simulink model "Kal_6Dpitch_sim"  (R2023b)
settings: Solver=FixedStepAuto  StartTime=0.0  StopTime=30  FixedStep=0.001  RelTol=1e-3
values from neighbouring files (symbols this model uses):
  beta = pi/10    (= 0.314159265359)    [Kal_6Dpitch_mat.m]    (also in TestValori.m = -0.628318530718; TestVel.m = 0.523598775598)
  cov_ic = [10, 0 ... (first row only)    [KalPrep_mat.m]    (also in Kal_6Dpitch_mat.m = cov_ic * (1 + 2*rand); Kal_pitch_mat.m = cov_ic * (1 + 2*rand))
  des_vel = [0.1, 0, 0, 0]'    [Kal_6Dpitch_mat.m]    (also in Los_path_mat.m)
  eta1 = deg2rad(1)    [KalPrep_mat.m]    (also in Kal_6Dpitch_mat.m = 0.05; Kal_pitch_mat.m = 0.15)
  eta2 = 0.05    [Kal_6Dpitch_mat.m]    (also in Kal_pitch_mat.m = 0.2)
  G = [Ts 0 ... (first row only)    [KalPrep_mat.m]    (also in Kal_6Dpitch_mat.m = eye(3) * Ts; Kal_pitch_mat.m = eye(3) * Ts)
  Gamma = -pi/6    (= -0.523598775598)    [Kal_6Dpitch_mat.m]    (also in TestValori.m)
  h_ref = 7    [Kal_6Dpitch_mat.m]
  init_cond = [pi/2; 5]    [KalPrep_mat.m]    (also in Kal_6Dpitch_mat.m = [2; 0; 0]; Kal_pitch_mat.m = [0; 0; 0])
  Kd_dep = (p + 2*damp*wn)*mv(3) + dv(3)    [Control_gains_mat.m]    (also in Los_path_mat.m = (p + 2*damp*wn)*mv(4) + dv(4))
  Ki_dep = p*(wn^2)*mv(3)    [Control_gains_mat.m]    (also in Los_path_mat.m = p*(wn^2)*mv(4))
  Ki_surge = wn^2 * mv(1)    [Control_gains_mat.m]    (also in Los_path_mat.m)
  Kp_dep = mv(3)*((wn^2) + 2*damp*p*wn)    [Control_gains_mat.m]    (also in Los_path_mat.m = mv(4)*((wn^2) + 2*damp*p*wn))
  Kp_surge = 2*damp*wn*mv(1) - dv(1)    [Control_gains_mat.m]    (also in Los_path_mat.m)
  Kt_dep = 1 / sqrt(ti_dep*td_dep)    [Control_gains_mat.m]
  Kt_surge = 1 / ti_surge    [Control_gains_mat.m]
  Lambda = pi/6    (= 0.523598775598)    [Kal_6Dpitch_mat.m]    (also in TestValori.m)
  pr0 = [0,0]'    [Kal_6Dpitch_mat.m]
  Q = [(sig1^2), 0 ... (first row only)    [KalPrep_mat.m]    (also in Kal_6Dpitch_mat.m = zeros(3,3); Kal_pitch_mat.m = zeros(3,3))
  qt = - 10    (= -10)    [Kal_6Dpitch_mat.m]    (also in TestValori.m = -5)
  R = (eta1)^2    [KalPrep_mat.m]    (also in Kal_6Dpitch_mat.m = [(eta1^2), 0; Kal_pitch_mat.m = [eta1, 0; untitled.m = 10)
  sat_dep = 15    [Model_6Deq_mat.m]
  sat_surge = 15    [Model_6Deq_mat.m]
  sat_tr = 2000    [Model_6Deq_mat.m]
  sig1 = 0.1    [KalPrep_mat.m]    (also in Kal_6Dpitch_mat.m; Kal_pitch_mat.m)
  sig2 = 0.2    [KalPrep_mat.m]    (also in Kal_6Dpitch_mat.m; Kal_pitch_mat.m)
  sig3 = 0.15    [Kal_6Dpitch_mat.m]    (also in Kal_pitch_mat.m)
  speed0 = [0.1, 0, 0, 0]'    [Los_path_mat.m]    (also in Model_6Deq_mat.m = [0.1, 0, 0, 0, 0, 0]')
  Ts = 0.001    [KalPrep_mat.m]    (also in Kal_6Dpitch_mat.m; Kal_pitch_mat.m; TestVel.m)
undefined symbols (not defined in the file or in its folder): Kd_theta, Ki_theta, Kp_theta, Kt_theta
settings Model: NumberOfSteps=100  SnapshotInterval=1000  Creator=fabio  LastModifiedBy=fabio

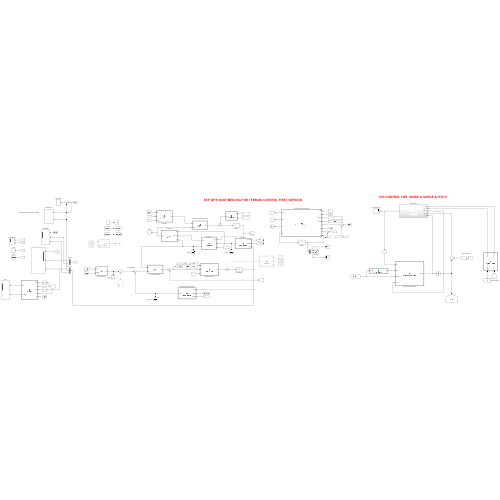
[thumbnail: Simulink's stored preview of the top-level diagram]
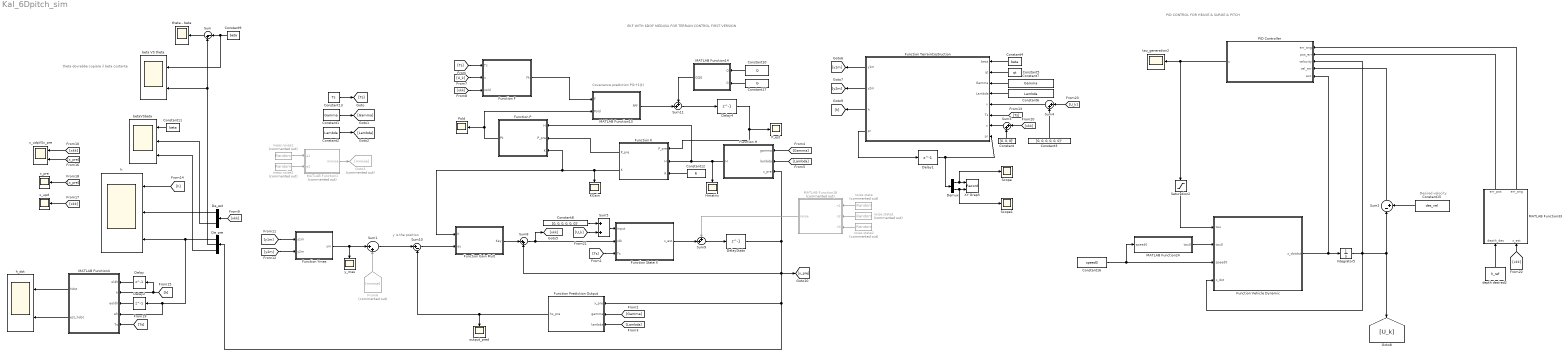
== system Kal_6Dpitch_sim ==
  note: theta dovrebbe copiare il beta costante
  note: Covariance prediction P(k+1|k)
  note: EKF WITH 6DOF MEDUSA FOR TERRAIN CONTROL FIRST VERSION
  note: y is the position
  note: PID CONTROL FOR HEAVE & SURGE & PITCH
  note: Desired velocity
  Constant : Constant  Value=[0, 0, 0]'
  Constant1 : Constant  Value=Gamma
  Constant10 : Constant  Value=Q  VectorParams1D=off
  Constant11 : Constant  Value=beta
  Constant12 : Constant  Value=R
  Constant13 : Constant  Value=Ts
  Constant15 : Constant  Value=des_vel
  Constant16 : Constant  Value=speed0
  Constant17 : Constant  Value=G  VectorParams1D=off
  Constant2 : Constant  Value=Lambda
  Constant3 : Constant  Value=[0, 0, 0, 0, 0, 0]'
  Constant4 : Constant  Value=beta
  Constant5 : Constant  Value=qt
  Constant6 : Constant  Value=Lambda
  Constant7 : Constant  Value=Gamma
  Constant8 : Constant  Value=[0, 0, 0, 0, 0, 0]'
  Constant9 : Constant  Value=beta
  De_est : Demux  Outputs=3
  De_pre : Demux  Outputs=3
  Delay : Delay  DelayLength=1
  Delay1 : Delay  DelayLength=1  InitialCondition=pr0  UseCircularBuffer=on
  Delay2 : Delay  DelayLength=1
  Delay4 : Delay  DelayLength=1  InitialCondition=cov_ic  UseCircularBuffer=on
  DelayStato : Delay  DelayLength=1  InitialCondition=init_cond  UseCircularBuffer=on
  Demux : Demux  Outputs=2
  From6 : From  Commented=on  GotoTag=mnoise
  Function F : MATLAB Function  TreatAsAtomicUnit=on
  Function Gain Mult : MATLAB Function  TreatAsAtomicUnit=on
  Function H : MATLAB Function  TreatAsAtomicUnit=on
  Function K : MATLAB Function  TreatAsAtomicUnit=on
  Function P : MATLAB Function  TreatAsAtomicUnit=on
  Function Prediction Output : MATLAB Function  TreatAsAtomicUnit=on
  Function State X : MATLAB Function  TreatAsAtomicUnit=on
  Function TerrainCostruction : MATLAB Function  TreatAsAtomicUnit=on
  Function Vehicle Dynamic : MATLAB Function  TreatAsAtomicUnit=on
  Function Ymes : MATLAB Function  TreatAsAtomicUnit=on
  Goto3 : Goto  Commented=on  GotoTag=mnoise
  Hmatrix : Scope
  Integrator5 : Integrator
  KGain : Scope
  MATLAB Function1 : MATLAB Function  Commented=on  TreatAsAtomicUnit=on
  MATLAB Function13 : MATLAB Function  TreatAsAtomicUnit=on
  MATLAB Function14 : MATLAB Function  TreatAsAtomicUnit=on
  MATLAB Function18 : MATLAB Function  Commented=on  TreatAsAtomicUnit=on
  MATLAB Function24 : MATLAB Function  TreatAsAtomicUnit=on
  MATLAB Function33 : MATLAB Function  TreatAsAtomicUnit=on
  MATLAB Function4 : MATLAB Function  TreatAsAtomicUnit=on
  PID Controller : Subsystem
  P_est : Scope
  Pold : Scope
  Saturation2 : Saturate  UpperLimit=sat_tr  LowerLimit=-sat_tr
  Scope : Scope
  Scope1 : Scope
  Sum : Sum  Inputs=|-+
  Sum{1,3..4,8} (4 alike) : Sum  Inputs=|++
  Sum10 : Sum  Inputs=|+-
  Sum11 : Sum  Inputs=++|
  Sum2 : Sum  Inputs=|-+
  Sum5 : Sum
  Sum9 : Sum  Inputs=++|
  XY Graph : Record  FileSettingsInternal="{\"entries\":[{\"content\":{\"excelSettings\":{\"content\":{},\"type\":\"Streamout.ExcelSettings\"}},\"type\":\"Streamout.FileSettingStorage\",\"uuid\":\"\"}],\"packageUris\":[\"http:\\/\\/schema.mathworks.com\\/mf0\\/streamout_blocks\\/R2020a\"],\"version\":\"1.0\"}"  Layout=[1 1]  SignalsInternal="{\"entries\":[{\"content\":{\"signals\":[{\"content\":{\"blockPath\":[],\"dimensions\":[1],\"domain\":\"\",\"lineColor\":\"#a2142f\",\"plots\":[ 1 ],\"port\":1,\"signalID\":1,\"signalName\":\"Demux:1\"},\"type\":\"RecordBlkView.Signal\",\"uuid\":\"\"},{\"content\":{\"blockPath\":[],\"dimensions\":[1],\"domain\":\"\",\"lineColor\":\"#139fff\",\"plots\":[ 1 ],\"port\":2,\"signalID\":2,\"signalName\":\"Demux:2\"},\"type\":\"RecordBlkView.Signal\",\"uuid\":\"\"}]},\"type\":\"RecordBlkView.InputSignals\",\"uuid\":\"\"}],\"packageUris\":[\"http:\\/\\/schema.mathworks.com\\/mf0\\/streamout_blocks\\/R2020a\"],\"version\":\"1.0\"}"  VisualizationBindings="{\"xyplotplugin\":{\"info\":[{\"series\":[{\"bindingParametersList\":[{\"parameter\":\"X-Axis\",\"signalID\":1,\"signalName\":\"Demux:1\"},{\"parameter\":\"Y-Axis\",\"signalID\":2,\"signalName\":\"Demux:2\"}],\"seriesID\":0}],\"subplotID\":1}]}}"  CompatibilityTag=XY
  beta VS theta : Scope  NumInputPorts=2
  betaVSbeta : Scope  NumInputPorts=3
  depth desired2 : Constant  Value=h_ref
  h : Scope  NumInputPorts=3
  h_dot : Scope  NumInputPorts=2
  meas.noise1 : RandomNumber  Commented=on  Variance=eta1  SampleTime=Ts
  meas.noise2 : RandomNumber  Commented=on  Variance=eta2  SampleTime=Ts
  noise state : RandomNumber  Commented=on  Variance=sig1  SampleTime=Ts
  noise state1 : RandomNumber  Commented=on  Variance=sig2  SampleTime=Ts
  noise state2 : RandomNumber  Commented=on  Variance=sig3  SampleTime=Ts
  output_pred : Scope
  tau_generation2 : Scope
  theta - beta : Scope
  x_pre : Scope
  x_udpVSx_pre : Scope  NumInputPorts=2
  x_upd : Scope
  y_mes : Scope
  wires:
  Function F/1(Fk) -> MATLAB Function13/1(F)
  DelayStato/1 -> Sum8/2, [x_pre], Function Prediction Output/1(x_pre), De_pre/1, Function H/3(x_pre)
  Delay4/1 -> P_est/1, Function K/1("P_pre ")
  Function Prediction Output/1(hx_pre) -> Sum10/2, output_pred/1
  Sum10/1 -> Function Gain Mult/2(ey)
  Function H/1(H) -> Hmatrix/1, Function P/1(H), Function K/2(H)
  Constant17/1 -> MATLAB Function14/2(G)
  MATLAB Function14/1(GQG) -> Sum11/1
  MATLAB Function13/1(FPF) -> Sum11/2
  Constant10/1 -> MATLAB Function14/1(Q)
  Function State X/1(x_est) -> Sum9/2
  Function P/1(Pk) -> Pold/1, MATLAB Function13/2(Pold)
  Sum9/1 -> DelayStato/1
  Constant12/1 -> Function K/3(R)
  Function K/2(K) -> KGain/1, Function P/3(K), Function Gain Mult/1(K)
  Sum11/1 -> Delay4/1
  Sum8/1 -> Function State X/2(xkk), [xkk]
  Function K/1(P_pre) -> Function P/2(P_pre)
  Function Gain Mult/1(Key) -> Sum8/1
  Function Ymes/1(ym) -> y_mes/1, Sum1/1
  Constant13/1 -> [Ts]
  [Ts] -> Function F/1(Ts)
  [Ts] -> Function State X/3(Ts)
  Constant1/1 -> [Gamma]
  Constant2/1 -> [Lambda]
  [Gamma] -> Function Prediction Output/2(gamma)
  [Lambda] -> Function Prediction Output/3(lambda)
  [Gamma] -> Function H/1(gamma)
  [Lambda] -> Function H/2(lambda)
  noise state/1 -> MATLAB Function18/1(n1)
  noise state2/1 -> MATLAB Function18/3(n3)
  noise state1/1 -> MATLAB Function18/2(n2)
  MATLAB Function18/1(noise) -> Sum9/1
  Sum1/1 -> Sum10/1
  meas.noise1/1 -> MATLAB Function1/1(e1)
  meas.noise2/1 -> MATLAB Function1/2(e2)
  MATLAB Function1/1(mnoise) -> Goto3/1
  [U_k] -> Function F/2(u)
  [xkk] -> Function F/3(xold)
  Delay1/1 -> Demux/1, Function TerrainCostruction/8("pr ")
  Function TerrainCostruction/4(pr) -> Delay1/1
  Function TerrainCostruction/1(y1m) -> [y1m]
  Function TerrainCostruction/2(y2m) -> [y2m]
  [y1m] -> Function Ymes/1(y1m)
  [y2m] -> Function Ymes/2(y2m)
  Constant4/1 -> Function TerrainCostruction/1(beta)
  Constant5/1 -> Function TerrainCostruction/2(qt)
  Constant6/1 -> Function TerrainCostruction/4(Lambda)
  [Ts] -> Function TerrainCostruction/6(Ts)
  Function TerrainCostruction/3(h) -> [h]
  [h] -> h/1
  [xkk] -> De_est/1
  De_est/1 -> h/2
  De_pre/1 -> MATLAB Function4/4(eh), Delay2/1, h/3
  Constant7/1 -> Function TerrainCostruction/3(Gamma)
  MATLAB Function4/1(hdot) -> h_dot/1
  De_est/3 -> betaVSbeta/2
  De_pre/3 -> betaVSbeta/3
  Constant11/1 -> betaVSbeta/1
  MATLAB Function4/2(est_hdot) -> h_dot/2
  [h] -> Delay/1, MATLAB Function4/2(h)
  Delay/1 -> MATLAB Function4/1(oldh)
  Delay2/1 -> MATLAB Function4/3(eoldh)
  [Ts] -> MATLAB Function4/5(Ts)
  From6/1 -> Sum1/2
  MATLAB Function24/1(tau0) -> Function Vehicle Dynamic/2(tau0)
  Constant16/1 -> Function Vehicle Dynamic/3(speed0), MATLAB Function24/1(speed0)
  Sum2/1 -> PID Controller/4(vel_err)
  PID Controller/1(u) -> tau_generation2/1, Saturation2/1
  MATLAB Function33/1(err_pos) -> PID Controller/2(pos_err)
  Function Vehicle Dynamic/1(x_dotdot) -> Integrator5/1, PID Controller/5(acc)
  Saturation2/1 -> Function Vehicle Dynamic/1(tau)
  depth desired2/1 -> MATLAB Function33/1(depth_des)
  Integrator5/1 -> PID Controller/3(velocity), Function Vehicle Dynamic/4(x_dot), [U_k], Sum2/1
  [xkk] -> MATLAB Function33/2(x_est)
  MATLAB Function33/2(err_ang) -> PID Controller/1(err_ang)
  Constant15/1 -> Sum2/2
  Constant9/1 -> beta VS theta/1, Sum/1
  Sum/1 -> theta - beta/1
  De_pre/2 -> beta VS theta/2, Sum/2
  [xkk] -> Sum3/1
  Sum3/1 -> Function TerrainCostruction/7(x)
  Constant/1 -> Sum3/2
  Sum4/1 -> Function TerrainCostruction/5(v)
  [U_k] -> Sum4/1
  Constant3/1 -> Sum4/2
  Demux/1 -> Scope/1, XY Graph/1
  Demux/2 -> Scope1/1, XY Graph/2
  Sum5/1 -> Function State X/1(input)
  Constant8/1 -> Sum5/1
  [U_k] -> Sum5/2
  [xkk] -> x_udpVSx_pre/1
  [xkk] -> x_upd/1
  [x_pre] -> x_pre/1
  [x_pre] -> x_udpVSx_pre/2

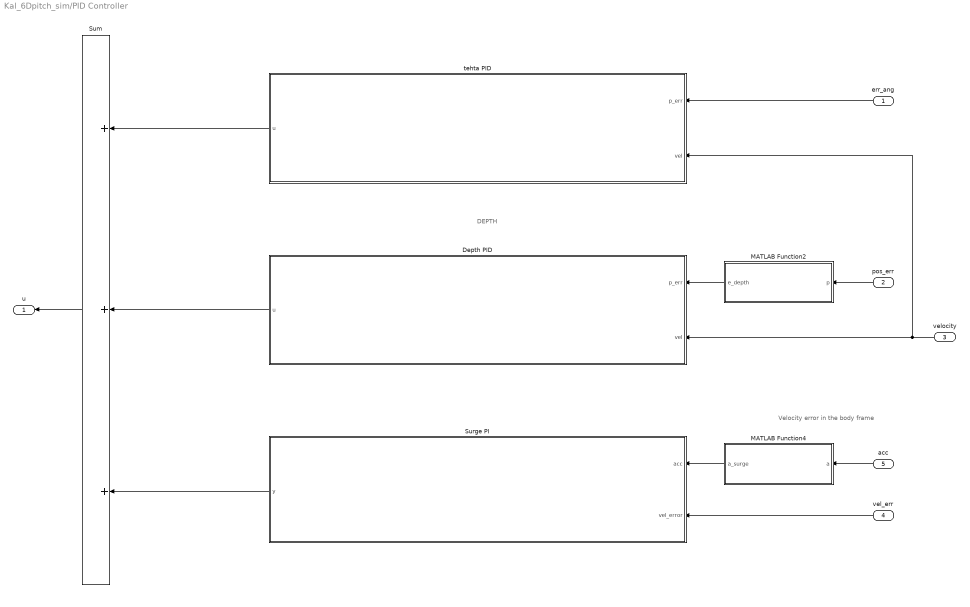
== system Kal_6Dpitch_sim/PID Controller ==
  note: Velocity error in the body frame
  note: DEPTH
  err_ang : Inport
  pos_err : Inport  Port=2
  velocity : Inport  Port=3
  vel_err : Inport  Port=4
  acc : Inport  Port=5
  Depth PID : Subsystem
  MATLAB Function2 : MATLAB Function  TreatAsAtomicUnit=on
  MATLAB Function4 : MATLAB Function  TreatAsAtomicUnit=on
  Sum : Sum  Inputs=+++
  Surge PI : Subsystem
  tehta PID : Subsystem
  u : Outport
  wires:
  velocity/1 -> Depth PID/2(vel), tehta PID/2(vel)
  vel_err/1 -> Surge PI/2(vel_error)
  MATLAB Function4/1(a_surge) -> Surge PI/1(acc)
  acc/1 -> MATLAB Function4/1(a)
  Surge PI/1(y) -> Sum/3
  Sum/1 -> u/1
  Depth PID/1(u) -> Sum/2
  pos_err/1 -> MATLAB Function2/1(p)
  MATLAB Function2/1(e_depth) -> Depth PID/1(p_err)
  tehta PID/1(u) -> Sum/1
  err_ang/1 -> tehta PID/1(p_err)

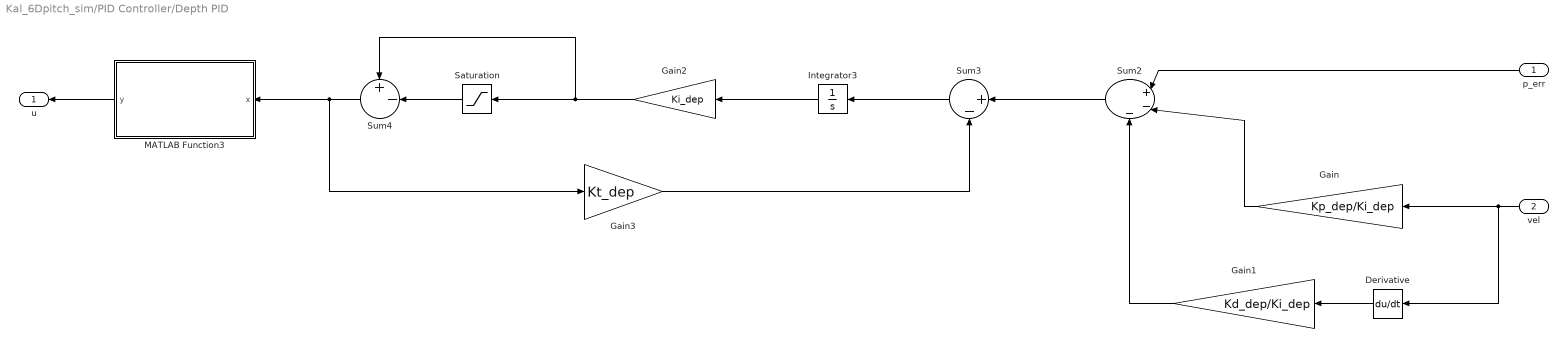
== system Kal_6Dpitch_sim/PID Controller/Depth PID ==
  p_err : Inport
  vel : Inport  Port=2
  Derivative : Derivative
  Gain : Gain  Gain=Kp_dep/Ki_dep
  Gain1 : Gain  Gain=Kd_dep/Ki_dep
  Gain2 : Gain  Gain=Ki_dep
  Gain3 : Gain  Gain=Kt_dep
  Integrator3 : Integrator
  MATLAB Function3 : MATLAB Function  TreatAsAtomicUnit=on
  Saturation : Saturate  UpperLimit=sat_dep  LowerLimit=-sat_dep
  Sum2 : Sum  Inputs=|+--
  Sum3 : Sum  Inputs=|+-
  Sum4 : Sum  Inputs=+-|
  u : Outport
  wires:
  Sum3/1 -> Integrator3/1
  Integrator3/1 -> Gain2/1
  Gain2/1 -> Sum4/1, Saturation/1
  Sum4/1 -> MATLAB Function3/1(x), Gain3/1
  Derivative/1 -> Gain1/1
  Saturation/1 -> Sum4/2
  Sum2/1 -> Sum3/1
  Gain/1 -> Sum2/2
  Gain1/1 -> Sum2/3
  p_err/1 -> Sum2/1
  vel/1 -> Derivative/1, Gain/1
  MATLAB Function3/1(y) -> u/1
  Gain3/1 -> Sum3/2

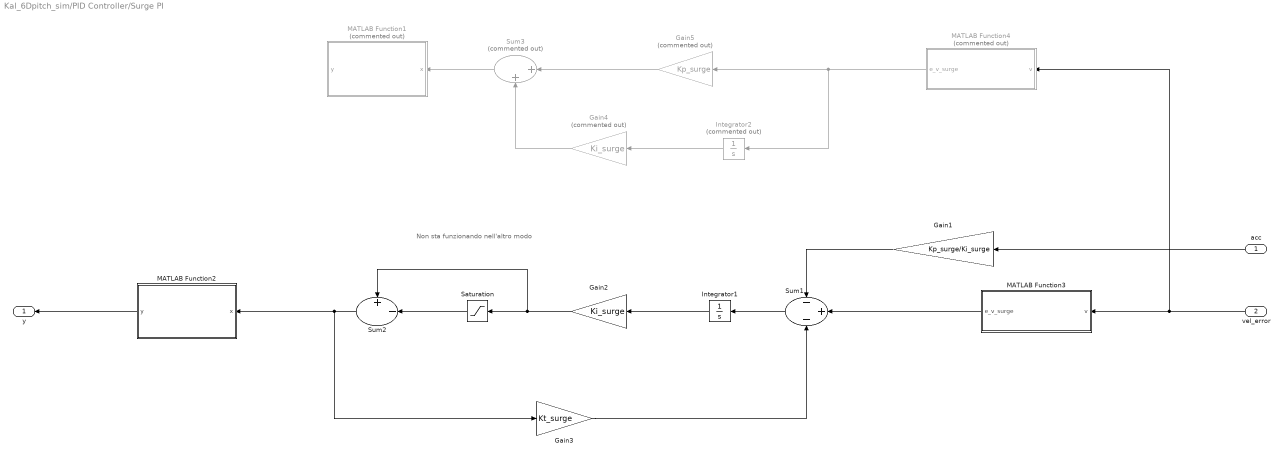
== system Kal_6Dpitch_sim/PID Controller/Surge PI ==
  note: Non sta funzionando nell'altro modo
  acc : Inport
  vel_error : Inport  Port=2
  Gain1 : Gain  Gain=Kp_surge/Ki_surge
  Gain2 : Gain  Gain=Ki_surge
  Gain3 : Gain  Gain=Kt_surge
  Gain4 : Gain  Commented=on  Gain=Ki_surge
  Gain5 : Gain  Commented=on  Gain=Kp_surge
  Integrator1 : Integrator
  Integrator2 : Integrator  Commented=on
  MATLAB Function1 : MATLAB Function  Commented=on  TreatAsAtomicUnit=on
  MATLAB Function2 : MATLAB Function  TreatAsAtomicUnit=on
  MATLAB Function3 : MATLAB Function  TreatAsAtomicUnit=on
  MATLAB Function4 : MATLAB Function  Commented=on  TreatAsAtomicUnit=on
  Saturation : Saturate  UpperLimit=sat_surge  LowerLimit=-sat_surge
  Sum1 : Sum  Inputs=-+-
  Sum2 : Sum  Inputs=+-|
  Sum3 : Sum  Commented=on  Inputs=|++
  y : Outport
  wires:
  Gain1/1 -> Sum1/1
  Sum2/1 -> Gain3/1, MATLAB Function2/1(x)
  Sum1/1 -> Integrator1/1
  Gain3/1 -> Sum1/3
  Saturation/1 -> Sum2/2
  Gain2/1 -> Sum2/1, Saturation/1
  Integrator1/1 -> Gain2/1
  MATLAB Function3/1(e_v_surge) -> Sum1/2
  Integrator2/1 -> Gain4/1
  vel_error/1 -> MATLAB Function3/1(v), MATLAB Function4/1(v)
  Gain5/1 -> Sum3/1
  Gain4/1 -> Sum3/2
  Sum3/1 -> MATLAB Function1/1(x)
  MATLAB Function4/1(e_v_surge) -> Integrator2/1, Gain5/1
  acc/1 -> Gain1/1
  MATLAB Function2/1(y) -> y/1

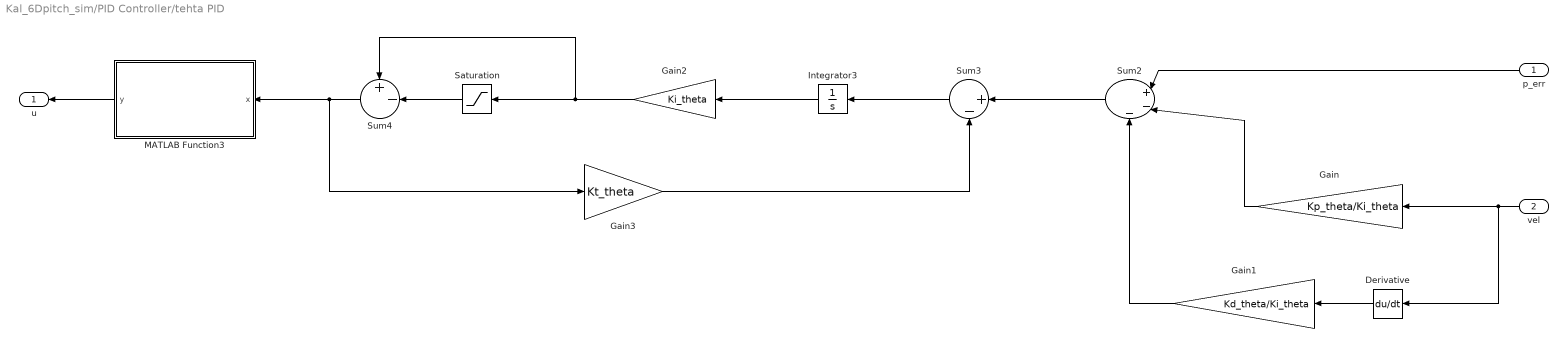
== system Kal_6Dpitch_sim/PID Controller/tehta PID ==
  p_err : Inport
  vel : Inport  Port=2
  Derivative : Derivative
  Gain : Gain  Gain=Kp_theta/Ki_theta
  Gain1 : Gain  Gain=Kd_theta/Ki_theta
  Gain2 : Gain  Gain=Ki_theta
  Gain3 : Gain  Gain=Kt_theta
  Integrator3 : Integrator
  MATLAB Function3 : MATLAB Function  TreatAsAtomicUnit=on
  Saturation : Saturate  UpperLimit=sat_dep  LowerLimit=-sat_dep
  Sum2 : Sum  Inputs=|+--
  Sum3 : Sum  Inputs=|+-
  Sum4 : Sum  Inputs=+-|
  u : Outport
  wires:
  Sum3/1 -> Integrator3/1
  Integrator3/1 -> Gain2/1
  Gain2/1 -> Sum4/1, Saturation/1
  Sum4/1 -> MATLAB Function3/1(x), Gain3/1
  Derivative/1 -> Gain1/1
  Saturation/1 -> Sum4/2
  Sum2/1 -> Sum3/1
  Gain/1 -> Sum2/2
  Gain1/1 -> Sum2/3
  p_err/1 -> Sum2/1
  vel/1 -> Derivative/1, Gain/1
  MATLAB Function3/1(y) -> u/1
  Gain3/1 -> Sum3/2

== matlab function Kal_6Dpitch_sim/MATLAB Function14 ==
  data: Q input; GQG output; G input
function GQG = GmatrixQ(Q, G)
    GQG = G*Q*(G');

== matlab function Kal_6Dpitch_sim/Function K ==
  data: P_pre output; P_pre input; H input; K output; R input
function [P_pre, K] = KalmanGain(P_pre, H, R)
    K = (P_pre*(H'))*pinv((H*P_pre*(H') + R));

== matlab function Kal_6Dpitch_sim/Function P ==
  data: H input; P_pre input; Pk output; K input
function Pk = PkComp(H ,P_pre, K)
    s = size((K*H), 1);
    I = eye(s); 
    Pk = (I - K*H)*P_pre;

== matlab function Kal_6Dpitch_sim/Function Gain Mult ==
  data: K input; ey input; Key output
function Key = GainMult(K, ey)
    Key = K*ey;

== matlab function Kal_6Dpitch_sim/Function F ==
  data: Fk output; Ts input; u input; xold input
function Fk = DynamicJacobian(Ts, u, xold)
    delta = xold(2) - xold(3);
    % u(1) = vsurge u, u(3) = vheave w, u(5) = q
    % !! ATTENZIONE:
    % STO CONSIDERANDO H RISPETTO TERRAIN FRAME E THETA E BETA RISPETTO
    % INERZIALE
    val = u(1)*cos(delta)+u(3)*sin(delta);
    F = [0, val, -val;
         0, 0, 0;
         0, 0, 0];
    Fk = eye(3) + Ts * F;

== matlab function Kal_6Dpitch_sim/MATLAB Function18 ==
  data: n1 input; n2 input; noise output; n3 input
function noise = StateNoise (n1, n2, n3)
    noise = [n1, n2, n3]';

== matlab function Kal_6Dpitch_sim/Function H ==
  data: gamma input; lambda input; x_pre input; H output
function H = HComputation(gamma, lambda, x_pre)
    % x(1) = h, x(2) = theta, x(3) = beta
    delta = [(gamma - (x_pre(3) - x_pre(2)));
             (lambda - (x_pre(3) - x_pre(2)))];

    val1 = (((x_pre(1)*sin(delta(1))) / ((cos(delta(1)))^2))) * sign(cos(delta(1)));
    val2 = (((x_pre(1)*sin(delta(2))) / ((cos(delta(2)))^2))) * sign(cos(delta(2)));

    H = [(1/abs(cos(delta(1)))), val1, -val1;
         (1/abs(cos(delta(2)))), val2, -val2];

== matlab function Kal_6Dpitch_sim/Function Ymes ==
  data: y1m input; y2m input; ym output
function ym = Ymeasured(y1m, y2m) 
    ym = [y1m; y2m];

== matlab function Kal_6Dpitch_sim/Function Vehicle Dynamic ==
  data: tau input; tau0 input; speed0 input; x_dot input; x_dotdot output
function x_dotdot = vehicle_dynamics_matrix(tau, tau0, speed0, x_dot)
    % updated to medusa model
    m = 11.5; % massa totale [kg]
    I = diag([0.21, 0.245, 0.245]);

    rho = 1028;
    volume = 0.011054;
    g = 9.81;

    % restoring
    z = 0.0420;
    B = rho * volume * g;


    % [surge, sway, heave, roll, pitch, yaw]
    % Added mass
    tau_a = [27.08; 25.952; 29.9081; 1; 1; 1]; % kl_dot 
    
    % Linear damping
    tau_r = [-0.1213; -1.1732; -1.1130; -0.5; -0.5; -0.5]; % linear_damping (kl)
    
    % Quadratic damping
    tau_d = [-23.9000; -46.2700; -50.2780; -1; -1; -1]; % quadratic_damping (kl_modl)
    
    % Virtual mass
    mv = [m; m; m; I(1,1); I(2,2); I(3,3)] - tau_a;
    
    % Dissipative forces (con v0 = 0.1 solo nel surge)
    dv = -tau_r - 2 * tau_d .* abs(speed0);

    delta = x_dot - speed0;

    % Accelerations
    % 6 DOF MODEL Linearized
    x_dotdot = zeros(6,1);
    tau(2) = 0;
    tau(4) = 0;
    
    % !! Attenzione queste sono equazioni lenearizzate attorno a un punto
    % di equilibrio e notevolmente semplificate -> da migliorare
    % surge
    x_dotdot(1) = (tau(1) - tau0(1) - dv(1)*delta(1)) / mv(1); % + mv(2)*speed0(2)*delta(6) + mv(2)*speed0(6)*delta(2)
    % sway
    x_dotdot(2) = (tau(2) - tau0(2) - dv(2)*delta(2)) / mv(2); % - mv(1)*speed0(1)*delta(6) - mv(1)*speed0(6)*delta(1)
    % heave
    x_dotdot(3) = (tau(3) - tau0(3) - dv(3)*delta(3)) / mv(3);
    % roll
    x_dotdot(4) = (tau(4) - tau0(4) - dv(4)*delta(4)) / mv(4);
    % pitch
    x_dotdot(5) = (tau(5) - tau0(5) - dv(5)*delta(5)) / mv(5);
    % yaw
    x_dotdot(6) = (tau(6) - tau0(6) - dv(6)*delta(6)) / mv(6); % + (mv(1) - mv(2))*speed0(1)*delta(2) + (mv(1) - mv(2))*speed0(2)*delta(1)
end

== matlab function Kal_6Dpitch_sim/MATLAB Function1 ==
  data: e1 input; e2 input; mnoise output
function mnoise = StateNoise (e1, e2)
    mnoise = [e1, e2]';

== matlab function Kal_6Dpitch_sim/MATLAB Function33 ==
  data: depth_des input; x_est input; err_pos output; err_ang output
function [err_pos, err_ang] = ErrorComputation(depth_des, x_est)
    err_pos = depth_des - x_est(1);
    err_ang = x_est(3) - x_est(2);
end

== matlab function Kal_6Dpitch_sim/PID Controller/Depth PID/MATLAB Function3 ==
  data: x input; y output
function y = Cond(x)
    y = zeros(6,1);
    y(3) = x(3);
end

== matlab function Kal_6Dpitch_sim/PID Controller/MATLAB Function4 ==
  data: a_surge output; a input
function a_surge  = Deviator(a)
    a_surge = a(1);
end

== matlab function Kal_6Dpitch_sim/PID Controller/Surge PI/MATLAB Function1 ==
  data: x input; y output
function y = Cond(x)
    y = zeros(4,1);
    y(1) = x;
end

== matlab function Kal_6Dpitch_sim/PID Controller/Surge PI/MATLAB Function2 ==
  data: x input; y output
function y = Cond(x)
    y = zeros(6,1);
    y(1) = x;
end

== matlab function Kal_6Dpitch_sim/PID Controller/Surge PI/MATLAB Function3 ==
  data: e_v_surge output; v input
function e_v_surge  = Deviator(v)
    e_v_surge = v(1);
end

== matlab function Kal_6Dpitch_sim/PID Controller/Surge PI/MATLAB Function4 ==
  data: e_v_surge output; v input
function e_v_surge  = Deviator(v)
    e_v_surge = v(1);
end

== matlab function Kal_6Dpitch_sim/Function TerrainCostruction ==
  data: beta input; qt input; y1m output; Gamma input; Lambda input; v input; Ts input; x input; y2m output; h output; pr input; pr output
function [y1m, y2m, h, pr] = MeasuramentComputation(beta, qt, Gamma, Lambda, v, Ts, x, pr) 
    % terrain construction
    mt = tan(beta);
    m1_g = tan((3*pi/2 + Gamma + x(2)));  
    m2_l = tan((3*pi/2 + Lambda + x(2)));

    % robot position on Matlab frame
    o_R_r = rotation(x(2));
    delta_p = o_R_r * [v(1), 0, v(3)]' * Ts;
    pr = pr + [delta_p(1), -delta_p(3)]';
    % line building equation   
    q1 = pr(2) - m1_g*pr(1);
    q2 = pr(2) - m2_l*pr(1);

    % computation for y1
    xc1 = (q1 - qt) / (mt - m1_g);
    yc1 = mt * xc1 + qt;
    y1m = norm([pr(1) - xc1; pr(2) - yc1]);

    % Computation for y2
    xc2 = (q2 - qt) / (mt - m2_l);
    yc2 = mt * xc2 + qt;
    y2m = norm([pr(1) - xc2; pr(2) - yc2]);
    
    % valore da ottenere di h
    h = (abs(mt*pr(1) - pr(2) + qt))/ (sqrt(mt^2 + 1));
end

function oRr = rotation(theta)
    roll = 0;
    yaw = 0;
    Rz = [cos(yaw), -sin(yaw), 0;
          sin(yaw), cos(yaw), 0;
          0, 0, 1];
    Ry = [cos(theta), 0, sin(theta);
          0, 1, 0;
          -sin(theta), 0, cos(theta)];
    Rx = [1 , 0, 0
          0, cos(roll), -sin(roll);
          0, sin(roll), cos(roll)];
    oRr = Rz*Ry*Rx;    
end

== matlab function Kal_6Dpitch_sim/MATLAB Function4 ==
  data: oldh input; h input; hdot output; eoldh input; eh input; Ts input; est_hdot output
function [hdot, est_hdot] =  Derivation(oldh, h, eoldh, eh, Ts)
    hdot = (h - oldh) / Ts;
    est_hdot = (eh - eoldh) / Ts;

== matlab function Kal_6Dpitch_sim/MATLAB Function24 ==
  data: tau0 output; speed0 input
function tau0 = tau0Computation(speed0)
    % updated to medusa model
    m = 11.5; % massa totale [kg]
    I = diag([0.21, 0.245, 0.245]);
    theta0 = 0;
    rho = 1028;
    volume = 0.011054;
    g = 9.81;

    % restoring
    z = 0.0420;
    B = rho * volume * g;
    

    % [surge, sway, heave, roll, pitch, yaw]
    % Added mass
    tau_a = [27.08; 25.952; 29.9081; 1; 1; 1]; % kl_dot 
    
    % Linear damping
    tau_r = [-0.1213; -1.1732; -1.1130; -0.5; -0.5; -0.5]; % linear_damping (kl)
    
    % Quadratic damping
    tau_d = [-23.9000; -46.2700; -50.2780; -1; -1; -1]; % quadratic_damping (kl_modl)
    
    % Virtual mass
    mv = [m; m; m; I(1,1); I(2,2); I(3,3)] - tau_a;

    % Dissatipative forces
    dv = -tau_r - 2*tau_d .* abs(speed0);
    
    % tau0 computation
    tau0 = zeros(6,1);
    tau0(1) = dv(1)*speed0(1); % - mv(2)*speed0(2)*speed0(4)
    tau0(2) = 0; % can do also the equations
    tau0(3) = dv(3)*speed0(3);
    % roll
    tau0(4) = 0;
    % pitch
    tau0(5) = dv(5)*speed0(5) + z*B*sin(theta0);
    % yaw
    tau0(6) = dv(6)*speed0(6); % - (mv(1) - mv(2))*speed0(1)*speed0(2)
    
end

== matlab function Kal_6Dpitch_sim/PID Controller/MATLAB Function2 ==
  data: p input; e_depth output
function e_depth  = Transformation(p)
    e_depth = - p;
end

== matlab function Kal_6Dpitch_sim/PID Controller/tehta PID/MATLAB Function3 ==
  data: x input; y output
function y = Cond(x)
    y = zeros(6,1);
    y(5) = x(5);
end

== matlab function Kal_6Dpitch_sim/Function State X ==
  data: input input; xkk input; x_est output; Ts input
function x_est = StatePrediction(input, xkk, Ts)
    % xkk(3) = beta, xkk(2) = theta
    % u(1) = vsurge, u(2) = vheave
    u = [input(1), input(3), input(5)]';
    A = eye(3);
    delta = xkk(2) - xkk(3);
    % considero h su seafloor frame
    B = [sin(delta), -cos(delta), 0;
         0, 0, 1;
         0, 0, 0];
    x_est = A*xkk + B*u*Ts;

== matlab function Kal_6Dpitch_sim/Function Prediction Output ==
  data: x_pre input; hx_pre output; gamma input; lambda input
function hx_pre = OutputPrediction(x_pre, gamma, lambda)
    delta = [(gamma - (x_pre(3) - x_pre(2)));
             (lambda - (x_pre(3) - x_pre(2)))];
    
    hx_pre = [x_pre(1)/abs((cos(delta(1))));
              x_pre(1)/abs((cos(delta(2))))];

== matlab function Kal_6Dpitch_sim/MATLAB Function13 ==
  data: F input; Pold input; FPF output
function FPF = FPFmatrix(F ,Pold)
    FPF = F*Pold*(F');
